simulink model "TFFuzzyComplete20Final"  (R2020b)
settings: Solver=FixedStepAuto  StartTime=0.0  StopTime=20  FixedStep=1e-3  RelTol=1e-1
InitFcn:
  | Param
values from neighbouring files (symbols this model uses):
  c = 3.5077E-3    (= 0.0035077)    [Param.m]
  d = 0.019    [Param.m]
  g = 9.81    [Param.m]
  J = (2/5)*m*r^2    (= 3.136704e-06)    [Param.m]
  Jm = 3.2284E-3    (= 0.0032284)    [Param.m]
  K = 0.0274    [Param.m]
  l = 0.118    [Param.m]
  L = 2.75E-3    (= 0.00275)    [Param.m]
  m = 0.051    [Param.m]
  R = 4    [Param.m]
  r = 0.0124    [Param.m]
libraries: simulink x4, fuzblock x2, pid_lib x2
settings Model: EnablePacing=on  PacingRate=316  Creator=HASSAN  LastModifiedBy=sara6
settings DebuggingCC: SFMachineParentedDataDiag=error

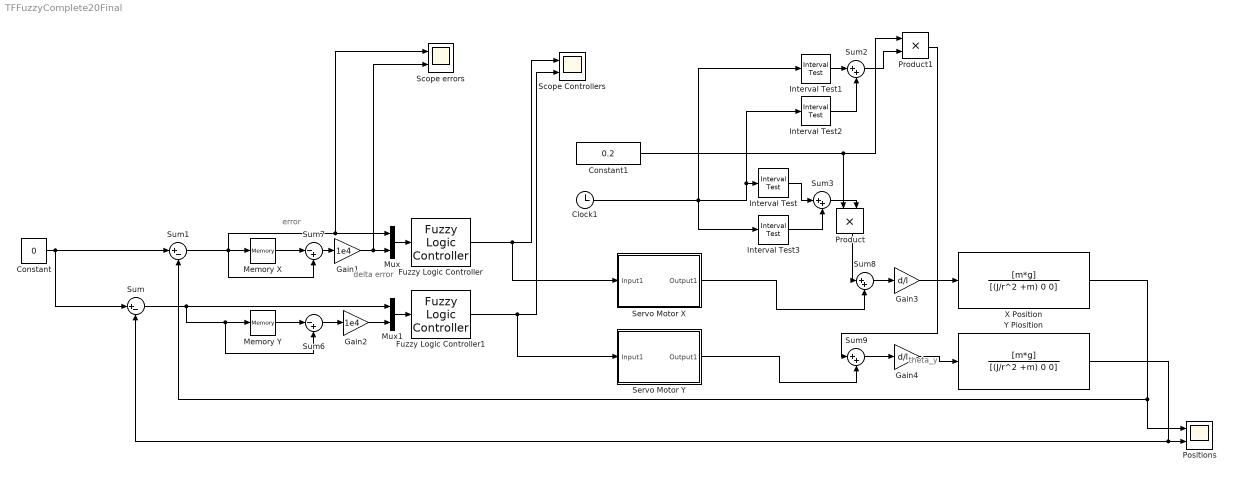
== system TFFuzzyComplete20Final ==
  note: delta error
  note: error
  note: theta_y
  Clock1 : Clock
  Constant : Constant  Value=0
  Constant1 : Constant  Value=0.2
  Fuzzy Logic Controller : fuzblock/Fuzzy Logic  Controller  FIS='simpleFuzzy.fis'  OutputSampleNumber=101  DataType=double  FuzzifiedInputs=off  RuleFiringStrengths=off  RuleOutputs=off  AggregatedOutputs=off  SimulateUsing=Code generation  OutOfRangeInputValueMessage=warning  NoRuleFiredMessage=warning  EmptyOutputFuzzySetMessage=warning
  Fuzzy Logic Controller1 : fuzblock/Fuzzy Logic  Controller  FIS='simpleFuzzy.fis'  OutputSampleNumber=101  DataType=double  FuzzifiedInputs=off  RuleFiringStrengths=off  RuleOutputs=off  AggregatedOutputs=off  SimulateUsing=Code generation  OutOfRangeInputValueMessage=warning  NoRuleFiredMessage=warning  EmptyOutputFuzzySetMessage=warning
  Gain1 : Gain  Gain=1e4
  Gain2 : Gain  Gain=1e4
  Gain3 : Gain  Gain=d/l
  Gain4 : Gain  Gain=d/l
  Interval Test : simulink/Logic and Bit Operations/Interval Test  IntervalClosedRight=on  uplimit=0.15  IntervalClosedLeft=on  lowlimit=0.1  OutDataTypeStr=boolean
  Interval Test1 : simulink/Logic and Bit Operations/Interval Test  IntervalClosedRight=on  uplimit=0.2  IntervalClosedLeft=on  lowlimit=0.1  OutDataTypeStr=boolean
  Interval Test2 : simulink/Logic and Bit Operations/Interval Test  IntervalClosedRight=on  uplimit=1.5  IntervalClosedLeft=on  lowlimit=1.3  OutDataTypeStr=boolean
  Interval Test3 : simulink/Logic and Bit Operations/Interval Test  IntervalClosedRight=on  uplimit=3  IntervalClosedLeft=on  lowlimit=2.6  OutDataTypeStr=boolean
  Memory X : Memory
  Memory Y : Memory
  Mux : Mux  Inputs=2
  Mux1 : Mux  Inputs=2
  Positions : Scope  NumInputPorts=2
  Product : Product
  Product1 : Product
  Scope Controllers : Scope  NumInputPorts=2
  Scope errors : Scope  NumInputPorts=2
  Servo Motor X : Subsystem
  Servo Motor Y : Subsystem
  Sum : Sum  Inputs=|+-
  Sum1 : Sum  Inputs=|+-
  Sum{2..3,8..9} (4 alike) : Sum  Inputs=|++
  Sum6 : Sum  Inputs=|-+
  Sum7 : Sum  Inputs=|-+
  X Position : TransferFcn  Numerator=[m*g]  Denominator=[(J/r^2 +m) 0 0]
  Y Piosition : TransferFcn  Numerator=[m*g]  Denominator=[(J/r^2 +m) 0 0]
  wires:
  Constant/1 -> Sum1/1, Sum/1
  Sum1/1 -> Memory X/1, Scope errors/1, Mux/1, Sum7/2
  X Position/1 -> Sum1/2, Positions/1
  Clock1/1 -> Interval Test1/1, Interval Test3/1, Interval Test2/1, Interval Test/1
  Sum/1 -> Mux1/1, Sum6/2, Memory Y/1
  Y Piosition/1 -> Sum/2, Positions/2
  Product1/1 -> Sum9/1
  Constant1/1 -> Product1/1, Product/1
  Interval Test1/1 -> Sum2/1
  Sum2/1 -> Product1/2
  Interval Test2/1 -> Sum2/2
  Interval Test/1 -> Sum3/1
  Interval Test3/1 -> Sum3/2
  Sum3/1 -> Product/2
  Memory Y/1 -> Sum6/1
  Memory X/1 -> Sum7/1
  Sum7/1 -> Gain1/1
  Gain1/1 -> Scope errors/2, Mux/2
  Gain2/1 -> Mux1/2
  Sum6/1 -> Gain2/1
  Gain3/1 -> X Position/1
  Product/1 -> Sum8/1
  Sum8/1 -> Gain3/1
  Gain4/1 -> Y Piosition/1
  Sum9/1 -> Gain4/1
  Mux/1 -> Fuzzy Logic Controller/1
  Mux1/1 -> Fuzzy Logic Controller1/1
  Fuzzy Logic Controller1/1 -> Servo Motor Y/1(Input1), Scope Controllers/2
  Fuzzy Logic Controller/1 -> Servo Motor X/1(Input1), Scope Controllers/1
  Servo Motor Y/1(Output1) -> Sum9/2
  Servo Motor X/1(Output1) -> Sum8/2

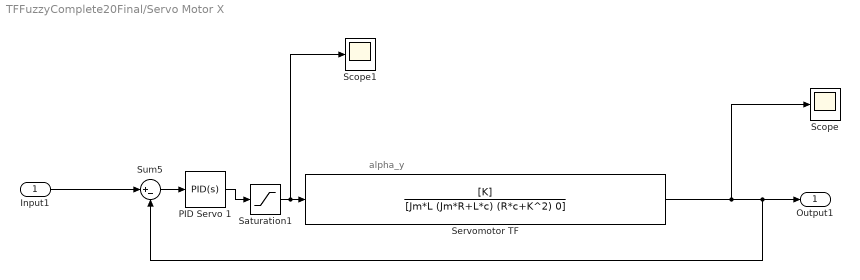
== system TFFuzzyComplete20Final/Servo Motor X ==
  note: alpha_y
  Input1 : Inport
  PID Servo 1 : pid_lib/PID Controller  Controller=PID  Form=Parallel  TimeDomain=Continuous-time  UseExternalTs=off  SampleTime=-1  IntegratorMethod=Forward Euler  FilterMethod=Forward Euler  ControllerParametersSource=internal  P=47.0508548732834  I=55.2080090820113  D=9.5699112835398  UseFilter=on  N=114.899439136233  TunerSelectOption=Transfer Function Based (PID Tuner App)  InitialConditionSource=internal  InitialConditionForIntegrator=0  InitialConditionForFilter=0  DifferentiatorICPrevScaledInput=0  ExternalReset=none  TrackingMode=off  Kt=1  LimitOutput=off  SatLimitsSource=internal  UpperSaturationLimit=inf  LowerSaturationLimit=-inf  LinearizeAsGain=on  AntiWindupMode=none  Kb=1  POutMin=[]  POutMax=[]  IOutMin=[]  IOutMax=[]  DOutMin=[]  DOutMax=[]  NOutMin=[]  NOutMax=[]  SumOutMin=[]  SumOutMax=[]  SaturationOutMin=[]  SaturationOutMax=[]  PParamMin=[]  PParamMax=[]  IParamMin=[]  IParamMax=[]  DParamMin=[]  DParamMax=[]  NParamMin=[]  NParamMax=[]  KbParamMin=[]  KbParamMax=[]  KtParamMin=[]  KtParamMax=[]  KbOutMin=[]  KbOutMax=[]  KtOutMin=[]  KtOutMax=[]  IntegratorOutMin=[]  IntegratorOutMax=[]  FilterOutMin=[]  FilterOutMax=[]  SumI1OutMin=[]  SumI1OutMax=[]  SumI2OutMin=[]  SumI2OutMax=[]  SumI3OutMin=[]  SumI3OutMax=[]  SumI4OutMin=[]  SumI4OutMax=[]  SumDOutMin=[]  SumDOutMax=[]  DifferentiatorOutMin=[]  DifferentiatorOutMax=[]  FilterDiffOutCoefMin=[]  FilterDiffOutCoefMax=[]  ReciprocalOutMin=[]  ReciprocalOutMax=[]  SumDenOutMin=[]  SumDenOutMax=[]  SumNumOutMin=[]  SumNumOutMax=[]  DivideOutMin=[]  DivideOutMax=[]  UdiffTsProdOutMin=[]  UdiffTsProdOutMax=[]  NTsProdOutMin=[]  NTsProdOutMax=[]  UintegralTsProdOutMin=[]  UintegralTsProdOutMax=[]  UngainTsProdOutMin=[]  UngainTsProdOutMax=[]  IntegratorContinuousStateAttributes=''  IntegratorStateMustResolveToSignalObject=off  IntegratorRTWStateStorageClass=Auto  FilterContinuousStateAttributes=''  FilterStateMustResolveToSignalObject=off  FilterRTWStateStorageClass=Auto  ParallelPVariant=InternalParameters  IdealPVariant=Disabled  IVariant=InternalParameters  DVariant=InternalParameters  IntegratorVariant=Continuous  SatVariant=Disabled  AWVariant=Passthrough  PCopyVariant=Disabled  TRVariant=Disabled  FdbkBlocksVariant=Forward  IdealPFdbkVariant=Disabled  SatFdbkVariant=Disabled  DerivativeFilterVariant=ContFilter  NVariant=InternalParameters  NCopyVariant=Disabled  FilterICVariant=InternalICsFilter  IntegratorICVariant=InternalICs  ExternalResetVariant=Disabled  TRSumVariant=Passthrough  SumFdbkVariant=Disabled  SumVariant=Sum_PID  TsampFilterVariant=InternalTs  TsampNgainVariant=Passthrough  TsampIntegralVariant=Passthrough  ExternalSaturationOutDataTypeStr=Inherit: Same as second input
  Saturation1 : Saturate  UpperLimit=7.8  LowerLimit=-7.8
  Scope : Scope
  Scope1 : Scope
  Servomotor TF : TransferFcn  Numerator=[K]  Denominator=[Jm*L (Jm*R+L*c) (R*c+K^2) 0]
  Sum5 : Sum  Inputs=|+-
  Output1 : Outport
  wires:
  Sum5/1 -> PID Servo 1/1
  PID Servo 1/1 -> Saturation1/1
  Input1/1 -> Sum5/1
  Saturation1/1 -> Scope1/1, Servomotor TF/1
  Servomotor TF/1 -> Scope/1, Output1/1, Sum5/2

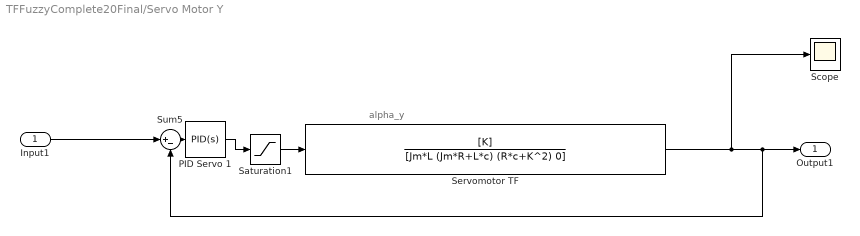
== system TFFuzzyComplete20Final/Servo Motor Y ==
  note: alpha_y
  Input1 : Inport
  PID Servo 1 : pid_lib/PID Controller  Controller=PID  Form=Parallel  TimeDomain=Continuous-time  UseExternalTs=off  SampleTime=-1  IntegratorMethod=Forward Euler  FilterMethod=Forward Euler  ControllerParametersSource=internal  P=47.0508548732834  I=55.2080090820113  D=9.5699112835398  UseFilter=on  N=114.899439136233  TunerSelectOption=Transfer Function Based (PID Tuner App)  InitialConditionSource=internal  InitialConditionForIntegrator=0  InitialConditionForFilter=0  DifferentiatorICPrevScaledInput=0  ExternalReset=none  TrackingMode=off  Kt=1  LimitOutput=off  SatLimitsSource=internal  UpperSaturationLimit=inf  LowerSaturationLimit=-inf  LinearizeAsGain=on  AntiWindupMode=none  Kb=1  POutMin=[]  POutMax=[]  IOutMin=[]  IOutMax=[]  DOutMin=[]  DOutMax=[]  NOutMin=[]  NOutMax=[]  SumOutMin=[]  SumOutMax=[]  SaturationOutMin=[]  SaturationOutMax=[]  PParamMin=[]  PParamMax=[]  IParamMin=[]  IParamMax=[]  DParamMin=[]  DParamMax=[]  NParamMin=[]  NParamMax=[]  KbParamMin=[]  KbParamMax=[]  KtParamMin=[]  KtParamMax=[]  KbOutMin=[]  KbOutMax=[]  KtOutMin=[]  KtOutMax=[]  IntegratorOutMin=[]  IntegratorOutMax=[]  FilterOutMin=[]  FilterOutMax=[]  SumI1OutMin=[]  SumI1OutMax=[]  SumI2OutMin=[]  SumI2OutMax=[]  SumI3OutMin=[]  SumI3OutMax=[]  SumI4OutMin=[]  SumI4OutMax=[]  SumDOutMin=[]  SumDOutMax=[]  DifferentiatorOutMin=[]  DifferentiatorOutMax=[]  FilterDiffOutCoefMin=[]  FilterDiffOutCoefMax=[]  ReciprocalOutMin=[]  ReciprocalOutMax=[]  SumDenOutMin=[]  SumDenOutMax=[]  SumNumOutMin=[]  SumNumOutMax=[]  DivideOutMin=[]  DivideOutMax=[]  UdiffTsProdOutMin=[]  UdiffTsProdOutMax=[]  NTsProdOutMin=[]  NTsProdOutMax=[]  UintegralTsProdOutMin=[]  UintegralTsProdOutMax=[]  UngainTsProdOutMin=[]  UngainTsProdOutMax=[]  IntegratorContinuousStateAttributes=''  IntegratorStateMustResolveToSignalObject=off  IntegratorRTWStateStorageClass=Auto  FilterContinuousStateAttributes=''  FilterStateMustResolveToSignalObject=off  FilterRTWStateStorageClass=Auto  ParallelPVariant=InternalParameters  IdealPVariant=Disabled  IVariant=InternalParameters  DVariant=InternalParameters  IntegratorVariant=Continuous  SatVariant=Disabled  AWVariant=Passthrough  PCopyVariant=Disabled  TRVariant=Disabled  FdbkBlocksVariant=Forward  IdealPFdbkVariant=Disabled  SatFdbkVariant=Disabled  DerivativeFilterVariant=ContFilter  NVariant=InternalParameters  NCopyVariant=Disabled  FilterICVariant=InternalICsFilter  IntegratorICVariant=InternalICs  ExternalResetVariant=Disabled  TRSumVariant=Passthrough  SumFdbkVariant=Disabled  SumVariant=Sum_PID  TsampFilterVariant=InternalTs  TsampNgainVariant=Passthrough  TsampIntegralVariant=Passthrough  ExternalSaturationOutDataTypeStr=Inherit: Same as second input
  Saturation1 : Saturate  UpperLimit=7.8  LowerLimit=-7.8
  Scope : Scope
  Servomotor TF : TransferFcn  Numerator=[K]  Denominator=[Jm*L (Jm*R+L*c) (R*c+K^2) 0]
  Sum5 : Sum  Inputs=|+-
  Output1 : Outport
  wires:
  Servomotor TF/1 -> Sum5/2, Output1/1, Scope/1
  Saturation1/1 -> Servomotor TF/1
  Input1/1 -> Sum5/1
  PID Servo 1/1 -> Saturation1/1
  Sum5/1 -> PID Servo 1/1
